simulink model "vsi"  (R2024b)
settings: Solver=VariableStepAuto  StartTime=0.0  StopTime=.2  RelTol=1e-3
values from neighbouring files (symbols this model uses):
  c = 1/(((wc)^2)*l)    (= 3.01551141793e-06)    [vsi_codes.m]
  f_op = 50    [vsi_codes.m]
  l = 8.4e-3    (= 0.0084)    [vsi_codes.m]
  m = .4    (= 0.4)    [vsi_codes.m]
  r = ((vop_rms)^2)/p_op    (= 52.9)    [vsi_codes.m]
  v3dc = 2*sqrt(2)*v3op_phaserms/m    [vsi_codes.m]
  vi_dc = ((vop_rms)*sqrt(2))/m    [vsi_codes.m]
libraries: spsIGBTDiodeLib x14, spsSeriesRLCBranchLib x6, spsDCVoltageSourceLib x3, spsThreePhaseSeriesRLCBranchLib x3, spsTriangleGeneratorLib x3, spsMultimeterLib x2, spsThreePhaseVIMeasurementLib x2, spsVoltageMeasurementLib x2, spsGroundLib x1, sps_lib x1
settings Model: Creator=91798  LastModifiedBy=91798

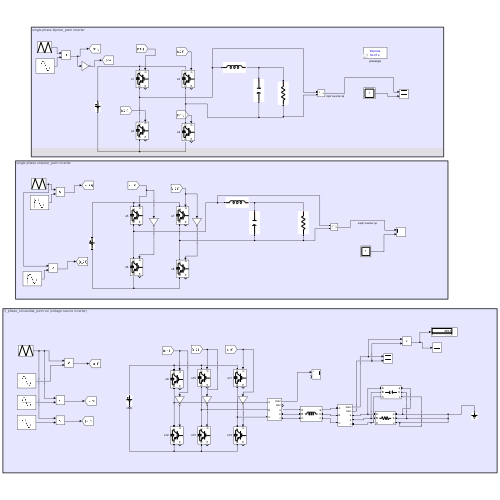
[thumbnail: Simulink's stored preview of the top-level diagram]
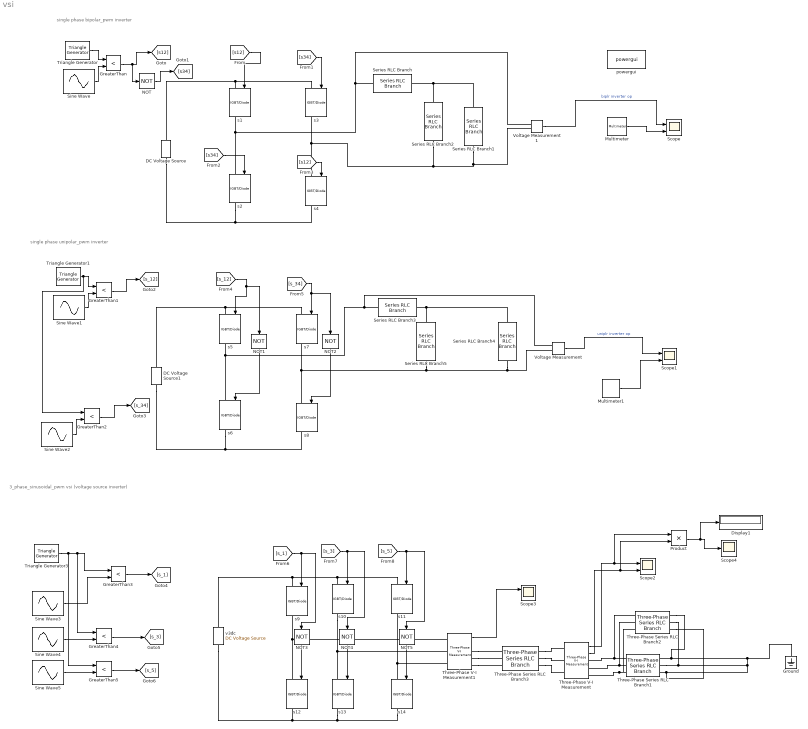
== system vsi ==
  note: single phase bipolar_pwm inverter
  note: single phase unipolar_pwm inverter
  note: 3_phase_sinusoidal_pwm vsi (voltage source inverter)
  DC Voltage Source : spsDCVoltageSourceLib/DC Voltage Source  Amplitude=vi_dc  Measurements=None
  DC Voltage Source1 : spsDCVoltageSourceLib/DC Voltage Source  Amplitude=vi_dc  Measurements=None
  Display1 : Display
  GreaterThan{,1..5} (6 alike) : RelationalOperator  Operator=<  OutDataTypeStr=boolean  RndMeth=Simplest  InputSameDT=off
  Ground : spsGroundLib/Ground  LConnTagsString=a
  Multimeter : spsMultimeterLib/Multimeter  L=2  sel=1  yselected={}  Gain=1  OutputType=Complex  PlotAtSimulationStop=off  PhasorSimulation=off
  Multimeter1 : spsMultimeterLib/Multimeter  L=2  sel=2  yselected={}  Gain=1  OutputType=Complex  PlotAtSimulationStop=off  PhasorSimulation=off
  NOT{,1..5} (6 alike) : Logic  Operator=NOT  IconShape=distinctive  AllPortsSameDT=off  OutDataTypeStr=boolean
  Product : Product
  Scope{,1..3} (4 alike) : Scope  NumInputPorts=2
  Scope4 : Scope
  Series RLC Branch : spsSeriesRLCBranchLib/Series RLC Branch  LConnTagsString=__new0  RConnTagsString=__new0  BranchType=L  Resistance=1  Inductance=l  SetiL0=off  InitialCurrent=0  Capacitance=1e-6  Setx0=off  InitialVoltage=0  Measurements=None
  Series RLC Branch1 : spsSeriesRLCBranchLib/Series RLC Branch  LConnTagsString=__new0  RConnTagsString=__new0  BranchType=R  Resistance=r  Inductance=1e-3  SetiL0=off  InitialCurrent=0  Capacitance=1e-6  Setx0=off  InitialVoltage=0  Measurements=Branch voltage
  Series RLC Branch2 : spsSeriesRLCBranchLib/Series RLC Branch  LConnTagsString=__new0  RConnTagsString=__new0  BranchType=C  Resistance=1  Inductance=1e-3  SetiL0=off  InitialCurrent=0  Capacitance=c  Setx0=off  InitialVoltage=0  Measurements=None
  Series RLC Branch3 : spsSeriesRLCBranchLib/Series RLC Branch  LConnTagsString=__new0  RConnTagsString=__new0  BranchType=L  Resistance=1  Inductance=l  SetiL0=off  InitialCurrent=0  Capacitance=1e-6  Setx0=off  InitialVoltage=0  Measurements=None
  Series RLC Branch4 : spsSeriesRLCBranchLib/Series RLC Branch  LConnTagsString=__new0  RConnTagsString=__new0  BranchType=R  Resistance=r  Inductance=1e-3  SetiL0=off  InitialCurrent=0  Capacitance=1e-6  Setx0=off  InitialVoltage=0  Measurements=Branch voltage
  Series RLC Branch5 : spsSeriesRLCBranchLib/Series RLC Branch  LConnTagsString=__new0  RConnTagsString=__new0  BranchType=C  Resistance=1  Inductance=1e-3  SetiL0=off  InitialCurrent=0  Capacitance=c  Setx0=off  InitialVoltage=0  Measurements=None
  Sine Wave : Sin  Amplitude=m  Frequency=f_op  SampleTime=0
  Sine Wave1 : Sin  Amplitude=m  Frequency=f_op  SampleTime=0
  Sine Wave2 : Sin  Amplitude=m  Frequency=f_op  Phase=pi  SampleTime=0
  Sine Wave3 : Sin  Amplitude=m  Frequency=f_op  SampleTime=0
  Sine Wave4 : Sin  Amplitude=m  Frequency=f_op  Phase=2*pi/3  SampleTime=0
  Sine Wave5 : Sin  Amplitude=m  Frequency=f_op  Phase=-2*pi/3  SampleTime=0
  Three-Phase Series RLC Branch1 : spsThreePhaseSeriesRLCBranchLib/Three-Phase Series RLC Branch  LConnTagsString=A|B|C  RConnTagsString=A|B|C  BranchType=R  Resistance=28.5  Inductance=l  Capacitance=1e-6  Measurements=None
  Three-Phase Series RLC Branch2 : spsThreePhaseSeriesRLCBranchLib/Three-Phase Series RLC Branch  LConnTagsString=A|B|C  RConnTagsString=A|B|C  BranchType=C  Resistance=r  Inductance=l  Capacitance=c  Measurements=None
  Three-Phase Series RLC Branch3 : spsThreePhaseSeriesRLCBranchLib/Three-Phase Series RLC Branch  LConnTagsString=A|B|C  RConnTagsString=A|B|C  BranchType=L  Resistance=r  Inductance=l  Capacitance=1e-6  Measurements=None
  Three-Phase V-I Measurement : spsThreePhaseVIMeasurementLib/Three-Phase V-I Measurement  VoltageMeasurement=phase-to-ground  SetLabelV=off  LabelV=Vabc  Vpu=off  VpuLL=off  CurrentMeasurement=yes  SetLabelI=off  LabelI=Iabc  Ipu=off  Pbase=100e6  Vbase=500e3  OutputType=Complex  PhasorSimulation=off  PSBequivalent=0
  Three-Phase V-I Measurement1 : spsThreePhaseVIMeasurementLib/Three-Phase V-I Measurement  VoltageMeasurement=phase-to-ground  SetLabelV=off  LabelV=Vabc  Vpu=off  VpuLL=off  CurrentMeasurement=yes  SetLabelI=off  LabelI=Iabc  Ipu=off  Pbase=100e6  Vbase=500e3  OutputType=Complex  PhasorSimulation=off  PSBequivalent=0
  Triangle Generator : spsTriangleGeneratorLib/Triangle Generator  Freq=fsw  Phase=0  Ts=0
  Triangle Generator1 : spsTriangleGeneratorLib/Triangle Generator  Freq=fsw  Phase=0  Ts=0
  Triangle Generator3 : spsTriangleGeneratorLib/Triangle Generator  Freq=fsw  Phase=0  Ts=0
  Voltage Measurement : spsVoltageMeasurementLib/Voltage Measurement  PhasorSimulation=off  OutputType=Complex  PSBequivalent=0
  Voltage Measurement1 : spsVoltageMeasurementLib/Voltage Measurement  PhasorSimulation=off  OutputType=Complex  PSBequivalent=0
  powergui : sps_lib/powergui  Priority=1  SimulationMode=Discrete  SampleTime=50e-8  frequency=60  Iterations=50  frequencyindice=0  Pbase=100e6  ErrMax=1e-4  UnitsV=kV  UnitsW=MW  buscounter=0  FunctionMessages=off  echomessages=off  EnableUseOfTLC=off  CurrentSourceSwitches=off  DisableSnubberDevices=off  DisableRonSwitches=off  DisableVfSwitches=off  DisplayEquations=off  AutomaticDiscreteSolvers=off  SolverType=Tustin/Backward Euler (TBE)  Interpol=off  ExternalGateDelay=off  methode=off  Ts=100  x0status=blocks  SPID=on  SwTol=0  HookPort=off  NonlinearTolerance=1e-4  nMaxIteration=100  ContinueOnMaxIteration=off  RestoreLinks=warning  ResistiveCurrentMeasurement=off  Frange=[0:2:500]  Ylog=off  Xlog=on  ShowGrid=off  save=off  variable=ZData  structure=0  ZoomFFT=off  StartTime=0.0  cycles=1  DisplayStyle=1  fundamental=60  FreqAxis=off  MaxFrequency=1000  frequencyindicesteady=1  RmsSteady=1  display=off
  s{1..14} (14 alike) : spsIGBTDiodeLib/IGBT//Diode  Ron=1e-3  Rs=1e5  Cs=inf  Measurements=on
  v3dc : spsDCVoltageSourceLib/DC Voltage Source  Amplitude=v3dc  Measurements=None
  wires:
  Triangle Generator/1 -> GreaterThan/1
  Sine Wave/1 -> GreaterThan/2
  GreaterThan/1 -> NOT/1, [s12]
  NOT/1 -> [s34]
  [s12] -> s1/1
  [s34] -> s3/1
  [s34] -> s2/1
  [s12] -> s4/1
  Multimeter/1 -> Scope/2
  NOT1/1 -> s6/1
  NOT2/1 -> s8/1
  Sine Wave1/1 -> GreaterThan1/2
  [s_34] -> NOT2/1, s7/1
  GreaterThan1/1 -> [s_12]
  [s_12] -> NOT1/1, s5/1
  Triangle Generator1/1 -> GreaterThan2/1, GreaterThan1/1
  Sine Wave2/1 -> GreaterThan2/2
  GreaterThan2/1 -> [s_34]
  Voltage Measurement/1 -> Scope1/1  "uniplr inverter op"
  Voltage Measurement1/1 -> Scope/1  "biplr inverter op"
  Multimeter1/1 -> Scope1/2
  [s_1] -> s9/1, NOT3/1
  [s_3] -> s10/1, NOT4/1
  [s_5] -> NOT5/1, s11/1
  NOT3/1 -> s12/1
  NOT4/1 -> s13/1
  NOT5/1 -> s14/1
  Triangle Generator3/1 -> GreaterThan5/1, GreaterThan4/1, GreaterThan3/1
  Sine Wave3/1 -> GreaterThan3/2
  Sine Wave4/1 -> GreaterThan4/2
  Sine Wave5/1 -> GreaterThan5/2
  GreaterThan3/1 -> [s_1]
  GreaterThan4/1 -> [s_3]
  GreaterThan5/1 -> [s_5]
  Three-Phase V-I Measurement/1 -> Product/1, Scope2/1
  Three-Phase V-I Measurement/2 -> Product/2, Scope2/2
  Three-Phase V-I Measurement1/1 -> Scope3/1
  Product/1 -> Display1/1, Scope4/1
  connections:
  s2/LConn1 -- Voltage Measurement1/LConn1 -- Series RLC Branch/RConn1 -- s1/RConn1
  s4/LConn1 -- Voltage Measurement1/LConn2 -- Series RLC Branch1/RConn1 -- Series RLC Branch2/RConn1 -- s3/RConn1
  s2/RConn1 -- DC Voltage Source/LConn1 -- s4/RConn1
  s1/LConn1 -- s3/LConn1 -- DC Voltage Source/RConn1
  Series RLC Branch1/LConn1 -- Series RLC Branch2/LConn1 -- Series RLC Branch/LConn1
  Series RLC Branch4/LConn1 -- Series RLC Branch3/LConn1 -- Series RLC Branch5/LConn1
  s8/LConn1 -- Voltage Measurement/LConn2 -- Series RLC Branch4/RConn1 -- Series RLC Branch5/RConn1 -- s7/RConn1
  s6/LConn1 -- Voltage Measurement/LConn1 -- Series RLC Branch3/RConn1 -- s5/RConn1
  s6/RConn1 -- DC Voltage Source1/LConn1 -- s8/RConn1
  s5/LConn1 -- s7/LConn1 -- DC Voltage Source1/RConn1
  s12/LConn1 -- Three-Phase V-I Measurement1/LConn1 -- s9/RConn1
  s10/RConn1 -- s13/LConn1 -- Three-Phase V-I Measurement1/LConn2
  s14/LConn1 -- Three-Phase V-I Measurement1/LConn3 -- s11/RConn1
  s10/LConn1 -- v3dc/RConn1 -- s9/LConn1 -- s11/LConn1
  v3dc/LConn1 -- s12/RConn1 -- s13/RConn1 -- s14/RConn1
  Three-Phase Series RLC Branch1/LConn1 -- Three-Phase Series RLC Branch2/LConn1 -- Three-Phase V-I Measurement/RConn1
  Three-Phase Series RLC Branch1/LConn2 -- Three-Phase V-I Measurement/RConn2 -- Three-Phase Series RLC Branch2/LConn2
  Three-Phase Series RLC Branch1/LConn3 -- Three-Phase V-I Measurement/RConn3 -- Three-Phase Series RLC Branch2/LConn3
  Three-Phase Series RLC Branch1/RConn3 -- Three-Phase Series RLC Branch1/RConn2 -- Three-Phase Series RLC Branch2/RConn2 -- Three-Phase Series RLC Branch2/RConn1 -- Three-Phase Series RLC Branch1/RConn1 -- Ground/LConn1 -- Three-Phase Series RLC Branch2/RConn3
  Three-Phase Series RLC Branch3/RConn1 -- Three-Phase V-I Measurement/LConn1
  Three-Phase Series RLC Branch3/RConn2 -- Three-Phase V-I Measurement/LConn2
  Three-Phase Series RLC Branch3/RConn3 -- Three-Phase V-I Measurement/LConn3
  Three-Phase V-I Measurement1/RConn1 -- Three-Phase Series RLC Branch3/LConn1
  Three-Phase V-I Measurement1/RConn2 -- Three-Phase Series RLC Branch3/LConn2
  Three-Phase V-I Measurement1/RConn3 -- Three-Phase Series RLC Branch3/LConn3
